simulink model "uni_model"  (R2017b)
settings: Solver=FixedStepAuto  StartTime=0.0  StopTime=20  FixedStep=dt  RelTol=1e-3
values from neighbouring files (symbols this model uses):
  dt = 0.1    [extendedKalmanFilter.m]    (also in matlab.mat; runV3.m; rungen.m; runpathfollower.m)
  i0 = 0    [matlab.mat]    (also in runV3.m = [0 0]')
  xi0 = [0 0 0 0 0 0 0 0]    [matlab.mat]    (also in runV3.m = [0 0 0 0 0 0 0 0]'; runpathfollower.m = [xi,yi,0,0,0,0,theta_mi,0]'; runpathplanner.m = [xi,yi,0,0,0,0,theta_mi,0]')
libraries: simulink x9
settings Model: Creator=nisha  LastModifiedBy=nisha

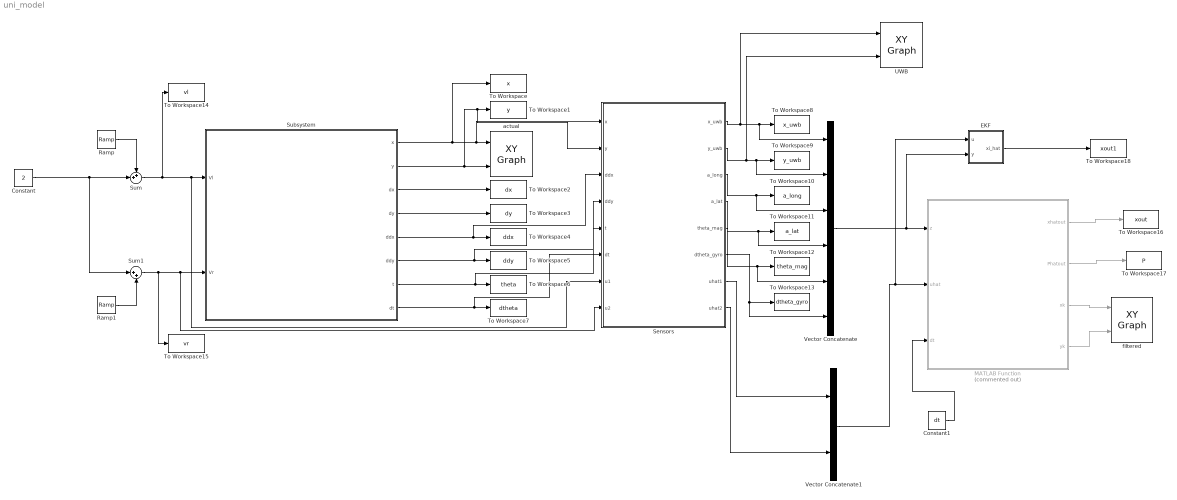
== system uni_model ==
  Constant : Constant  Value=2
  Constant1 : Constant  Value=dt
  EKF : Subsystem
  MATLAB Function : MATLAB Function  Commented=on  TreatAsAtomicUnit=on
  Ramp : simulink/Sources/Ramp  slope=0.1  start=2  X0=0
  Ramp1 : simulink/Sources/Ramp  slope=0.1  start=3  X0=0
  Sensors : Subsystem  Description=dfg
  Subsystem : Subsystem
  Sum : Sum  Inputs=++|
  Sum1 : Sum  Inputs=|++
  To Workspace : ToWorkspace  VariableName=x  SampleTime=-1
  To Workspace1 : ToWorkspace  VariableName=y  SampleTime=-1
  To Workspace10 : ToWorkspace  VariableName=a_long  SampleTime=-1
  To Workspace11 : ToWorkspace  VariableName=a_lat  SampleTime=-1
  To Workspace12 : ToWorkspace  VariableName=theta_mag  SampleTime=-1
  To Workspace13 : ToWorkspace  VariableName=dtheta_gyro  SampleTime=-1
  To Workspace14 : ToWorkspace  VariableName=vl  SampleTime=-1
  To Workspace15 : ToWorkspace  VariableName=vr  SampleTime=-1
  To Workspace16 : ToWorkspace  VariableName=xout  SampleTime=-1
  To Workspace17 : ToWorkspace  VariableName=P  SampleTime=-1
  To Workspace18 : ToWorkspace  VariableName=xout1  SampleTime=-1
  To Workspace2 : ToWorkspace  VariableName=dx  SampleTime=-1
  To Workspace3 : ToWorkspace  VariableName=dy  SampleTime=-1
  To Workspace4 : ToWorkspace  VariableName=ddx  SampleTime=-1
  To Workspace5 : ToWorkspace  VariableName=ddy  SampleTime=-1
  To Workspace6 : ToWorkspace  VariableName=theta  SampleTime=-1
  To Workspace7 : ToWorkspace  VariableName=dtheta  SampleTime=-1
  To Workspace8 : ToWorkspace  VariableName=x_uwb  SampleTime=-1
  To Workspace9 : ToWorkspace  VariableName=y_uwb  SampleTime=-1
  UWB : simulink/Sinks/XY Graph  xmin=-5  xmax=15  ymin=-15  ymax=10  st=-1
  Vector Concatenate : Concatenate  NumInputs=6
  Vector Concatenate1 : Concatenate
  actual : simulink/Sinks/XY Graph  xmin=-5  xmax=15  ymin=-15  ymax=10  st=-1
  filtered : simulink/Sinks/XY Graph  xmin=-5  xmax=15  ymin=-15  ymax=10  st=-1
  wires:
  Constant/1 -> Sum1/1, Sum/2
  Sum/1 -> To Workspace14/1, Sensors/7(u1), Subsystem/1(Vl)
  Ramp/1 -> Sum/1
  Ramp1/1 -> Sum1/2
  Subsystem/1(x) -> To Workspace/1, actual/1, Sensors/1(x)
  Subsystem/2(y) -> actual/2, Sensors/2(y), To Workspace1/1
  Subsystem/3(dx) -> To Workspace2/1
  Subsystem/4(dy) -> To Workspace3/1
  Subsystem/5(ddx) -> Sensors/3(ddx), To Workspace4/1
  Subsystem/6(ddy) -> Sensors/4(ddy), To Workspace5/1
  Subsystem/7(t) -> Sensors/5(t), To Workspace6/1
  Subsystem/8(dt) -> Sensors/6(dt), To Workspace7/1
  Sensors/1("x_uwb ") -> UWB/1, Vector Concatenate/1, To Workspace8/1
  Sensors/2(y_uwb) -> UWB/2, Vector Concatenate/2, To Workspace9/1
  Sensors/5(theta_mag) -> Vector Concatenate/5, To Workspace12/1
  Sensors/4(a_lat) -> Vector Concatenate/4, To Workspace11/1
  Sensors/6(dtheta_gyro) -> Vector Concatenate/6, To Workspace13/1
  Sensors/3(a_long) -> Vector Concatenate/3, To Workspace10/1
  Vector Concatenate/1 -> EKF/2(y), MATLAB Function/1(z)
  MATLAB Function/2(Phatout) -> To Workspace17/1
  MATLAB Function/1(xhatout) -> To Workspace16/1
  Constant1/1 -> MATLAB Function/3(dt)
  MATLAB Function/3(xk) -> filtered/1
  MATLAB Function/4(yk) -> filtered/2
  Vector Concatenate1/1 -> EKF/1(u), MATLAB Function/2(uhat)
  Sum1/1 -> To Workspace15/1, Sensors/8(u2), Subsystem/2(Vr)
  Sensors/7(uhat1) -> Vector Concatenate1/1
  Sensors/8(uhat2) -> Vector Concatenate1/2
  EKF/1(xi_hat) -> To Workspace18/1

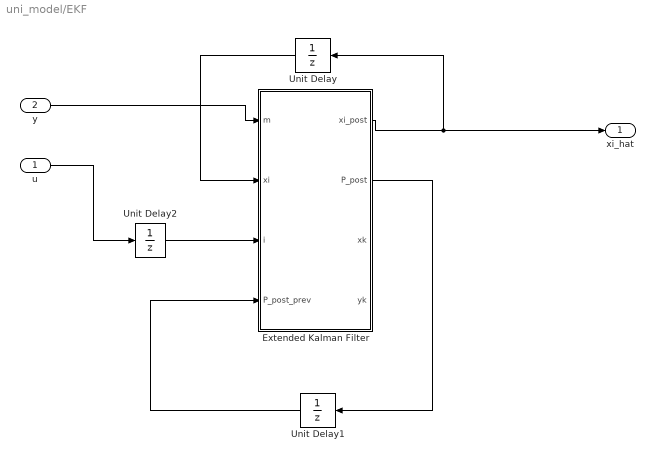
== system uni_model/EKF ==
  u : Inport
  y : Inport  Port=2
  Extended Kalman Filter : MATLAB Function  TreatAsAtomicUnit=on
  Unit Delay : UnitDelay  InitialCondition=xi0  SampleTime=-1
  Unit Delay1 : UnitDelay  InitialCondition=zeros(8,8)  SampleTime=-1
  Unit Delay2 : UnitDelay  InitialCondition=i0  SampleTime=-1
  xi_hat : Outport
  wires:
  Extended Kalman Filter/1(xi_post) -> xi_hat/1, Unit Delay/1
  y/1 -> Extended Kalman Filter/1(m)
  u/1 -> Unit Delay2/1
  Unit Delay2/1 -> Extended Kalman Filter/3(i)
  Unit Delay/1 -> Extended Kalman Filter/2(xi)
  Extended Kalman Filter/2(P_post) -> Unit Delay1/1
  Unit Delay1/1 -> Extended Kalman Filter/4(P_post_prev)

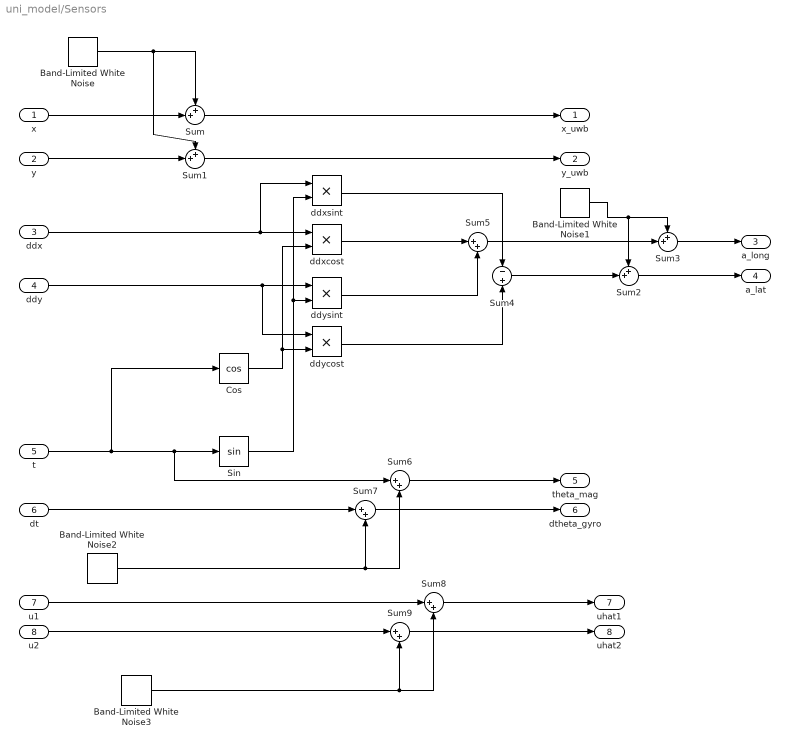
== system uni_model/Sensors ==
  x : Inport
  y : Inport  Port=2
  ddx : Inport  Port=3
  ddy : Inport  Port=4
  t : Inport  Port=5
  dt : Inport  Port=6
  u1 : Inport  Port=7
  u2 : Inport  Port=8
  Band-Limited White Noise : simulink/Sources/Band-Limited White Noise  Cov=0.1  Ts=dt  seed=[23341]
  Band-Limited White Noise1 : simulink/Sources/Band-Limited White Noise  Cov=0.01  Ts=dt  seed=[23341]
  Band-Limited White Noise2 : simulink/Sources/Band-Limited White Noise  Cov=0.001  Ts=dt  seed=[23341]
  Band-Limited White Noise3 : simulink/Sources/Band-Limited White Noise  Cov=0.0001  Ts=dt  seed=[23341]
  Cos : Trigonometry  Operator=cos
  Sin : Trigonometry
  Sum{,1..3} (4 alike) : Sum  Inputs=++|
  Sum4 : Sum  Inputs=-|+
  Sum{5..9} (5 alike) : Sum  Inputs=|++
  ddxcost : Product
  ddxsint : Product
  ddycost : Product
  ddysint : Product
  "x_uwb " : Outport
  y_uwb : Outport  Port=2
  a_long : Outport  Port=3
  a_lat : Outport  Port=4
  theta_mag : Outport  Port=5
  dtheta_gyro : Outport  Port=6
  uhat1 : Outport  Port=7
  uhat2 : Outport  Port=8
  wires:
  x/1 -> Sum/2
  y/1 -> Sum1/2
  Band-Limited White Noise/1 -> Sum1/1, Sum/1
  Sum/1 -> "x_uwb "/1
  Sum1/1 -> y_uwb/1
  Band-Limited White Noise1/1 -> Sum2/1, Sum3/1
  t/1 -> Sum6/1, Sin/1, Cos/1
  ddx/1 -> ddxcost/1, ddxsint/1
  Cos/1 -> ddxcost/2, ddycost/2
  Sin/1 -> ddxsint/2, ddysint/2
  ddy/1 -> ddycost/1, ddysint/1
  Sum5/1 -> Sum3/2
  Sum4/1 -> Sum2/2
  ddxcost/1 -> Sum5/1
  ddysint/1 -> Sum5/2
  ddxsint/1 -> Sum4/1
  ddycost/1 -> Sum4/2
  Sum6/1 -> theta_mag/1
  dt/1 -> Sum7/1
  Sum7/1 -> dtheta_gyro/1
  Band-Limited White Noise2/1 -> Sum7/2, Sum6/2
  Sum3/1 -> a_long/1
  Sum2/1 -> a_lat/1
  Band-Limited White Noise3/1 -> Sum8/2, Sum9/2
  Sum9/1 -> uhat2/1
  u2/1 -> Sum9/1
  Sum8/1 -> uhat1/1
  u1/1 -> Sum8/1

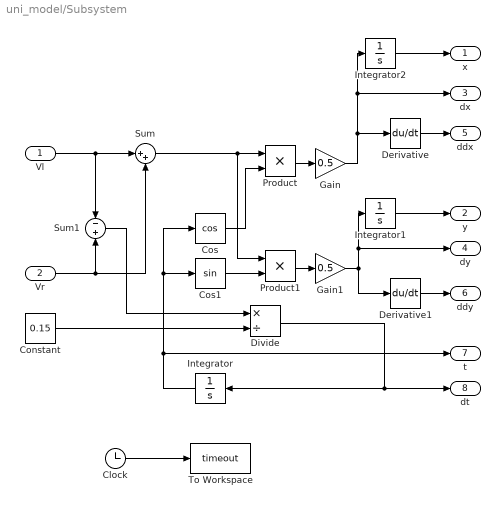
== system uni_model/Subsystem ==
  Vl : Inport
  Vr : Inport  Port=2
  Clock : Clock
  Constant : Constant  Value=0.15
  Cos : Trigonometry  Operator=cos
  Cos1 : Trigonometry
  Derivative : Derivative
  Derivative1 : Derivative
  Divide : Product  Inputs=*/
  Gain : Gain  Gain=0.5
  Gain1 : Gain  Gain=0.5
  Integrator : Integrator
  Integrator1 : Integrator
  Integrator2 : Integrator
  Product : Product
  Product1 : Product
  Sum : Sum  Inputs=|++
  Sum1 : Sum  Inputs=-|+
  To Workspace : ToWorkspace  VariableName=timeout  SaveFormat=Timeseries  SampleTime=-1
  x : Outport
  y : Outport  Port=2
  dx : Outport  Port=3
  dy : Outport  Port=4
  ddx : Outport  Port=5
  ddy : Outport  Port=6
  t : Outport  Port=7
  dt : Outport  Port=8
  wires:
  Vl/1 -> Sum/1, Sum1/1
  Vr/1 -> Sum/2, Sum1/2
  Sum/1 -> Product1/1, Product/1
  Product1/1 -> Gain1/1
  Product/1 -> Gain/1
  Gain1/1 -> Derivative1/1, Integrator1/1, dy/1
  Constant/1 -> Divide/2
  Divide/1 -> Integrator/1, dt/1
  Sum1/1 -> Divide/1
  Cos/1 -> Product/2
  Cos1/1 -> Product1/2
  Integrator/1 -> t/1, Cos1/1, Cos/1
  Integrator1/1 -> y/1
  Integrator2/1 -> x/1
  Gain/1 -> Derivative/1, Integrator2/1, dx/1
  Derivative/1 -> ddx/1
  Derivative1/1 -> ddy/1
  Clock/1 -> To Workspace/1

== matlab function uni_model/MATLAB Function ==
  settings: updateMethod=DISCRETE
  data: z input; xhatout output; uhat input; dt input; Phatout output; xk output; yk output
function [xhatout,Phatout,xk,yk] = extendedKalman(z,uhat,dt)
%   Implements an extended Kalman filter used for object tracking.

%   The states of the process are given by
%   x = [x_pos y_pos x_vel y_vel x_acc y_acc phi omega]^T
%   x = [x y dx dx ddx ddy theta dtheta]^T
%   Measurements given by 
%   z = [x_uwb y_uwb a_long a_lat theta_mag dtheta_gyro]^T
persistent P xhat R M Q
if isempty(P)
    %     Initiation
    xhat = [0;0;2;2;0;0;0;0];
    uhat = [0;0];
    
    P = zeros(8,8);
    Q = diag([0.1,0.1,0.1,0.1,0.1,0.1,0.1,0.1]);
    R = diag([0.001/dt, 0.001/dt, 0.01/dt, 0.01/dt, 0.001/dt, 0.001/dt]);
    M = diag([0.001, 0.001]);
%end
%P=initial.P; M=initial.M; R= initial.R; xhat=initial.x0;
end
d=0.15;
x=xhat(1,1); y=xhat(2,1); dx=xhat(3,1); dy=xhat(4,1); ddx=xhat(5,1); ddy=xhat(6,1); phik=xhat(7,1); dphi=xhat(8,1);
vl=uhat(1,1); vr=uhat(2,1);
% Calculate the Jacobians for the state and measurement equations
phi=phik + 1/2*dphi*dt;

        
xhat= [x + dt*dx + (ddx*dt^2)/2 + (dt*vl*cos(phi))/2 + (dt*vr*cos(phi))/2
 y + dt*dy + (ddy*dt^2)/2 + (dt*vl*sin(phi))/2 + (dt*vr*sin(phi))/2
                    dx + ddx*dt + (vl*cos(phi))/2 + (vr*cos(phi))/2
                    dy + ddy*dt + (vl*sin(phi))/2 + (vr*sin(phi))/2
                                                                ddx
                                                                ddy
                              (d*phi - dt*vl + dt*vr + d*dphi*dt)/d
                                               (vr - vl + d*dphi)/d];

% Jacobians
F =     [ 1, 0, dt,  0, dt^2/2,      0, -(dt*sin(phi)*(vl + vr))/2,  0
          0, 1,  0, dt,      0, dt^2/2,  (dt*cos(phi)*(vl + vr))/2,  0
          0, 0,  1,  0,     dt,      0,    -(sin(phi)*(vl + vr))/2,  0
          0, 0,  0,  1,      0,     dt,     (cos(phi)*(vl + vr))/2,  0
          0, 0,  0,  0,      1,      0,                          0,  0
          0, 0,  0,  0,      0,      1,                          0,  0
          0, 0,  0,  0,      0,      0,                          1, dt
          0, 0,  0,  0,      0,      0,                          0,  1];
V =     [ (dt*cos(phi))/2, (dt*cos(phi))/2
          (dt*sin(phi))/2, (dt*sin(phi))/2
               cos(phi)/2,      cos(phi)/2
               sin(phi)/2,      sin(phi)/2
                        0,               0
                        0,               0
                    -dt/d,            dt/d
                     -1/d,             1/d];
                                           
% Covariance update
P = F*P*F' + V*M*V' + Q;


% Measurement model

%   z = [x_uwb, y_uwb, a_long, a_lat, theta_mag, dtheta_gyro]^T
zhat = [1    0   0   0   0           0           0   0
     0    1   0   0   0           0           0   0
     0    0   0   0   cos(phi)    sin(phi)    0   0
     0    0   0   0   -sin(phi)   cos(phi)    0   0
     0    0   0   0   0           0           1   0
     0    0   0   0   0           0           0   1]*xhat;
 
% More Linearization
H = [ 1, 0, 0, 0,         0,        0,                             0, 0
      0, 1, 0, 0,         0,        0,                             0, 0
      0, 0, 0, 0,  cos(phi), sin(phi),   ddy*cos(phi) - ddx*sin(phi), 0
      0, 0, 0, 0, -sin(phi), cos(phi), - ddx*cos(phi) - ddy*sin(phi), 0
      0, 0, 0, 0,         0,        0,                             1, 0
      0, 0, 0, 0,         0,        0,                             0, 1];
  
% Calculate gain
K=P*H'/(H*P*H'+R);

%update
xhatout=xhat+K*(z-zhat);
Phatout=(1-K*H)*P;
xk=xhatout(1,1); yk=xhatout(2,1);
end

== matlab function uni_model/EKF/Extended Kalman Filter ==
  data: m input; xi input; i input; P_post_prev input; xi_post output; P_post output; xk output; yk output
function [xi_post,P_post,xk,yk] = fcn(m,xi,i,P_post_prev)
%% Prediction
% x = xi(1);      y     = xi(2);      z   = xi(3);
% u = xi(4);      v     = xi(5);      w   = xi(6);
% phi = xi(7);    theta = xi(8);      psi = xi(9);
% p   = xi(10);   q     = xi(11);     r   = xi(12);
% 
% tauphi = i(1);  tautheta = i(2);
% taupsi = i(3);  T = i(4);
d=0.15;
x=xi(1); y=xi(2); dx=xi(3); dy=xi(4); ddx=xi(5); ddy=xi(6); phi=xi(7); dphi=xi(8);
vl=i(1); vr=i(2);
dt=0.1;
xi_prio = ...
[x + dt*dx + (ddx*dt^2)/2 + (dt*vl*cos(phi))/2 + (dt*vr*cos(phi))/2
 y + dt*dy + (ddy*dt^2)/2 + (dt*vl*sin(phi))/2 + (dt*vr*sin(phi))/2
                    dx + ddx*dt + (vl*cos(phi))/2 + (vr*cos(phi))/2
                    dy + ddy*dt + (vl*sin(phi))/2 + (vr*sin(phi))/2
                                                                ddx
                                                                ddy
                              (d*phi - dt*vl + dt*vr + d*dphi*dt)/d
                                               (vr - vl + d*dphi)/d];

A = ...
[ 1, 0, dt,  0, dt^2/2,      0, -(dt*sin(phi)*(vl + vr))/2,  0
          0, 1,  0, dt,      0, dt^2/2,  (dt*cos(phi)*(vl + vr))/2,  0
          0, 0,  1,  0,     dt,      0,    -(sin(phi)*(vl + vr))/2,  0
          0, 0,  0,  1,      0,     dt,     (cos(phi)*(vl + vr))/2,  0
          0, 0,  0,  0,      1,      0,                          0,  0
          0, 0,  0,  0,      0,      1,                          0,  0
          0, 0,  0,  0,      0,      0,                          1, dt
          0, 0,  0,  0,      0,      0,                          0,  1];
Q = diag([0.1,0.1,0.1,0.1,0.1,0.1,0.1,0.1]);
P_prio = A*P_post_prev*A'+Q;

%% Update
zhat = [1    0   0   0   0           0           0   0
     0    1   0   0   0           0           0   0
     0    0   0   0   cos(phi)    sin(phi)    0   0
     0    0   0   0   -sin(phi)   cos(phi)    0   0
     0    0   0   0   0           0           1   0
     0    0   0   0   0           0           0   1]*xi_prio;
C =  [ 1, 0, 0, 0,         0,        0,                             0, 0;
      0, 1, 0, 0,         0,        0,                             0, 0;
      0, 0, 0, 0,  cos(phi), sin(phi),   ddy*cos(phi) - ddx*sin(phi), 0;
      0, 0, 0, 0, -sin(phi), cos(phi), - ddx*cos(phi) - ddy*sin(phi), 0;
      0, 0, 0, 0,         0,        0,                             1, 0;
      0, 0, 0, 0,         0,        0,                             0, 1];
  R = diag([0.001/dt, 0.001/dt, 0.01/dt, 0.01/dt, 0.001/dt, 0.001/dt]);
 K = P_prio*C'/(C*P_prio*C'+R);


% Update states and covariance matrix
xi_post = xi_prio + K*(m-zhat);
P_post = (eye(size(P_prio,1))-K*C)*P_prio*(eye(size(P_prio,1))-K*C)'+K*R*K';
xk=xi_post(1); yk=xi_post(2);
